simulink model "DSM5_2018a"  (R2018a)
settings: Solver=VariableStepAuto  StartTime=0.0  StopTime=0.6  RelTol=1e-3
settings Model: Creator=bzhan  LastModifiedBy=bzhan
settings DataIOCC: ReturnWorkspaceOutputs=on
settings SFSimCC: SimUseLocalCustomCode=on
settings RTWCC: RTWUseLocalCustomCode=on

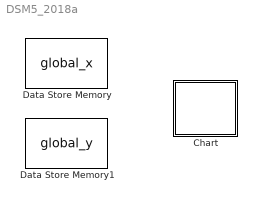
== system DSM5_2018a ==
  Chart : Stateflow chart  TreatAsAtomicUnit=on
  Data Store Memory : DataStoreMemory  DataStoreName=global_x  ReadBeforeWriteMsg=warning  WriteAfterWriteMsg=warning  WriteAfterReadMsg=warning  InitialValue=1  ShowAdditionalParam=off  OutDataTypeStr=int32
  Data Store Memory1 : DataStoreMemory  DataStoreName=global_y  ReadBeforeWriteMsg=warning  WriteAfterWriteMsg=warning  WriteAfterReadMsg=warning  InitialValue=2  ShowAdditionalParam=off  OutDataTypeStr=int32

== stateflow chart DSM5_2018a/Chart ==
  settings: updateMethod=DISCRETE  sampleTime=0.1
  state A
  state B
  (default) -> A : {v=global_y;
      |  global_x=global_x+v;}
  A -> B : {v=global_x+1;global_x=v;f()}
  B -> A : {v=global_y+2;global_y=v;f()}
  data: global_x data_store_memory; v local; global_y data_store_memory
  function f:
    | function f
    |   fprintf("%d %d\n", global_x, global_y);
